simulink model "MMC_Control_PLECS_IFB_diode_ab0"  (R2016a)
settings: Solver=VariableStepAuto  SolverMode=SingleTasking  StartTime=0.0  StopTime=0.02  FixedStep=sim_Ts  RelTol=1e-3
undefined symbols (not defined in the file or in its folder): plecs
settings Model: Creator=jason  LastModifiedBy=Francis Chen
settings DebuggingCC: SFUnexpectedBacktrackingDiag=error  SFNoUnconditionalDefaultTransitionDiag=error
settings SFSimCC: SimUseLocalCustomCode=on
settings RTWCC: RTWUseLocalCustomCode=on
settings GRTTargetCC: TargetLangStandard=C99 (ISO)  GeneratePreprocessorConditionals=Use local settings
settings ConfigComp: CovMetricSettings=dwe  CovHtmlReporting=off  CovSaveCumulativeToWorkspaceVar=off  CovSaveSingleToWorkspaceVar=off  CovExternalEMLEnable=on

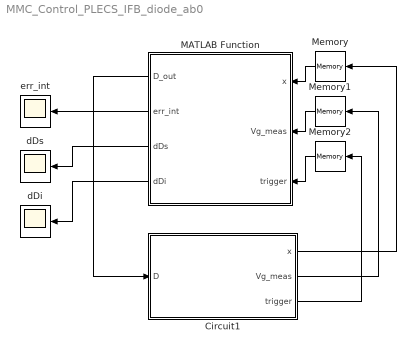
== system MMC_Control_PLECS_IFB_diode_ab0 ==
  Circuit1 : Subsystem  LoadFcn=plecs('sl', 200);  InitFcn=plecs('sl', 214);  StartFcn=plecs('sl', 208);  StopFcn=plecs('sl', 209);  mask(PlecsCircuit){PLECSData=<binary blob, 35032 chars, not shown>}
      mask prompts: PLECSData "PLECS Data (Do not delete or modify!)"
      mask init:
      | % PLACE CUSTOM INITIALIZATIONS ABOVE
      | % DO NOT REMOVE
      | plecs('sl', 215);
      | % DO NOT REMOVE
      settings: CopyFcn=plecs('sl', 203);  DeleteFcn=plecs('sl', 205);  UndoDeleteFcn=plecs('sl', 206);  PreSaveFcn=plecs('sl', 211);  PostSaveFcn=plecs('sl', 201);  NameChangeFcn=plecs('sl', 210);  DestroyFcn=plecs('sl', 207);  PreCopyFcn=plecs('sl', 216);  OpenFcn=plecs('sl', 202);  ErrorFcn=plerrorfcn
      mask Help: web(['file:///' fullfile(plecsdoc, 'creatingacircuit.html')])
      mask Display: disp('PLECS\nCircuit')
  MATLAB Function : MATLAB Function  TreatAsAtomicUnit=on
  Memory : Memory  X0=[50,50,50,4,4,4];  InheritSampleTime=on
  Memory1 : Memory  X0=[0,0,0];  InheritSampleTime=on
  Memory2 : Memory  InheritSampleTime=on
  dDi : Scope
  dDs : Scope
  err_int : Scope
  wires:
  Circuit1/3(trigger) -> Memory2/1
  Circuit1/2(Vg_meas) -> Memory1/1
  Circuit1/1(x) -> Memory/1
  MATLAB Function/1(D_out) -> Circuit1/1(D)
  Memory/1 -> MATLAB Function/1(x)
  Memory1/1 -> MATLAB Function/2(Vg_meas)
  Memory2/1 -> MATLAB Function/3(trigger)
  MATLAB Function/2(err_int) -> err_int/1
  MATLAB Function/3(dDs) -> dDs/1
  MATLAB Function/4(dDi) -> dDi/1

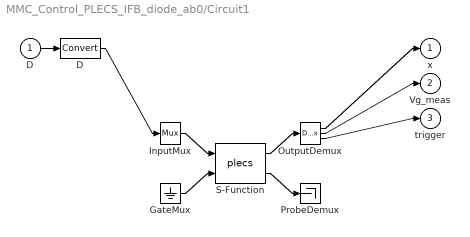
== system MMC_Control_PLECS_IFB_diode_ab0/Circuit1 ==
  D : Inport  PortDimensions=6
  " D " : DataTypeConversion  SaturateOnIntegerOverflow=on  RndMeth=Zero
  " GateMux " : Ground
  " InputMux " : Mux  Inputs=[ 6 ]
  " OutputDemux " : Demux  Outputs=[ 6 3 1 ]
  " ProbeDemux " : Terminator
  " S-Function " : S-Function  FunctionName=plecs  SFunctionDeploymentMode=off  EnableBusSupport=off
  x : Outport  PortDimensions=6
  Vg_meas : Outport  Port=2  PortDimensions=3
  trigger : Outport  Port=3  PortDimensions=1
  wires:
  " InputMux "/1 -> " S-Function "/1
  " GateMux "/1 -> " S-Function "/2
  " S-Function "/1 -> " OutputDemux "/1
  " S-Function "/2 -> " ProbeDemux "/1
  D/1 -> " D "/1
  " D "/1 -> " InputMux "/1
  " OutputDemux "/1 -> x/1
  " OutputDemux "/2 -> Vg_meas/1
  " OutputDemux "/3 -> trigger/1

== matlab function MMC_Control_PLECS_IFB_diode_ab0/MATLAB Function ==
  data: x input; D_out output; Vg_meas input; trigger input; nom parameter; err_int output; dDs output; dDi output
function [D_out,  err_int, dDs,dDi]= MMC_control_AB0(x, Vg_meas, trigger,nom)


persistent D_out_val err_int_val phi_val Di_out_val Ds_out_val
if isempty(D_out_val)
    phi_val = 0;
    D_out_val = [0.5; 0.5; 0.5; 0.5; 0.5; 0.5];
    Di_out_val = zeros(6,1); 
    Ds_out_val = zeros(6,1);
    err_int_val = zeros(5,1);
end

if trigger    
Vg_peak = 120; 
Lleak = 1e-6 ;
Nstate = 6; 
Nin  = 6; 
Nout = 5; 
Kclark = 2/3*[1,-0.5,-0.5;0 sqrt(3)/2 -sqrt(3)/2;1/3,1/3,1/3]; %clark transform for ABC 

sin_1     = (Vg_meas(1)/Vg_peak);
sin_2     = (Vg_meas(2)/Vg_peak); 
sin_3     = (Vg_meas(3)/Vg_peak); 

phi_1  = asin(sin_1); 
if (sin_1>=0) && (sin_2>=sin_3)
    phi_1 = pi-phi_1; 
end

if (sin_1<=0) && (sin_2>=sin_3) 
    phi_1 = pi-phi_1; 
end

if phi_1<0 
    phi_1 = phi_1+2*pi;  
end

phi = phi_1; 
tstep   = ceil(interp1(nom.phi,nom.id,phi,'nearest','extrap'));
xnom    = nom.x(tstep,:)'; 
% xnom(1:3) = [75 80 85]';% new setpoint

K       = nom.K(tstep,:,:);

xab       = [x(1:3);Kclark*x(4:6)]; %Clark Transformation to get the ab current
yab       = xab(1:5); 
yabd      = xnom(1:5); 

K  = reshape (K,Nstate,Nstate+Nout);
Ki = K       (:,1:Nout); 
Kp = K       (:,Nout+1:end);
tcy     = 1/nom.fsw;
D0      = nom.D (tstep,:)'; %Nominal Duty Cycle

state   =   xab - xnom; 
err     =   yabd - yab; 
err_int =   err*tcy  + err_int_val;

dD      = - Kp*state - Ki*err_int;
dDi     = -Ki*err_int; 
dDs     = -Kp*state;
D       =   D0+dD;  % pay close attention to the sign!
D       =   max(min(D,0.999),-0.999);

% convRatio = abs(D); 
% Dabs     = sqrt(convRatio); 
% D        = sign(D).*Dabs;
% R    = ones(1,Nin); 
% R(1) = x(1)*convRatio(1)/abs(x(4)); 
% R(2) = x(3)*convRatio(2)/abs(x(4)); 
% R(3) = x(1)*convRatio(3)/abs(x(5)); 
% R(4) = x(2)*convRatio(4)/abs(x(5)); 
% R(5) = x(2)*convRatio(5)/abs(x(6)); 
% R(6) = x(3)*convRatio(6)/abs(x(6));
% Dabs      = sqrt(convRatio.^2./(1-tcy*R./(4*Lleak*convRatio))); 

    D_out = D;
    Di_out_val = dDi; 
    Ds_out_val = dDs; 
    D_out_val = D;
    err_int_val = err_int;
    phi_val = phi; 
else
    phi = phi_val; 
    D_out = D_out_val;
    dDi  = Di_out_val; 
    dDs  = Ds_out_val; 
    err_int = err_int_val;
end

end %function
